simulink model "RlocusEx2"  (R2021a)
settings: Solver=VariableStepAuto  StartTime=0.0  StopTime=10.0  RelTol=1e-3
settings Model: Creator=User  LastModifiedBy=User

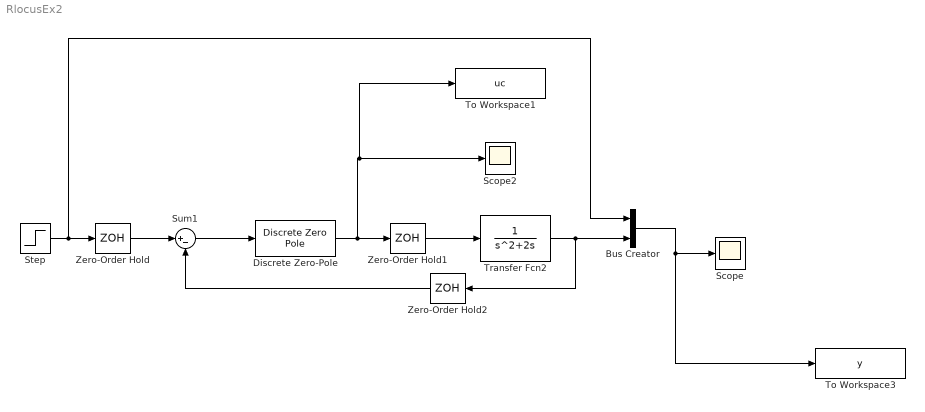
== system RlocusEx2 ==
  Bus Creator : BusCreator  Inputs=2
  Discrete Zero-Pole : DiscreteZeroPole  Zeros=[0.673]  Poles=[0.253]  Gain=12.659  SampleTime=-1
  Scope : Scope
  Scope2 : Scope
  Step : Step  SampleTime=0
  Sum1 : Sum  Inputs=|+-
  To Workspace1 : ToWorkspace  VariableName=uc  SaveFormat=Timeseries  SampleTime=-1
  To Workspace3 : ToWorkspace  VariableName=y  SaveFormat=Timeseries  SampleTime=-1
  Transfer Fcn2 : TransferFcn  Denominator=[1 2 0]
  Zero-Order Hold : ZeroOrderHold  SampleTime=0.2
  Zero-Order Hold1 : ZeroOrderHold  SampleTime=0.2
  Zero-Order Hold2 : ZeroOrderHold  SampleTime=0.2
  wires:
  Transfer Fcn2/1 -> Bus Creator/2, Zero-Order Hold2/1
  Zero-Order Hold2/1 -> Sum1/2
  Zero-Order Hold1/1 -> Transfer Fcn2/1
  Zero-Order Hold/1 -> Sum1/1
  Bus Creator/1 -> Scope/1, To Workspace3/1
  Step/1 -> Bus Creator/1, Zero-Order Hold/1
  Sum1/1 -> Discrete Zero-Pole/1
  Discrete Zero-Pole/1 -> To Workspace1/1, Scope2/1, Zero-Order Hold1/1
